simulink model "R0_to_Euler_Test"  (Simulink 7.5)
settings: Solver=ode45  StartTime=0.0  StopTime=10.0  RelTol=1e-3
values from neighbouring files (symbols this model uses):
  R0 = single(Euler2DCMdeg( PHI_IC, THETA_IC, PSI_IC ))    [demoz2SlugsV5.m]
libraries: SLUGS_Library x3, dspmtrx3 x1, simulink x1
settings Model: Creator=Robert  LastModifiedBy=Robert

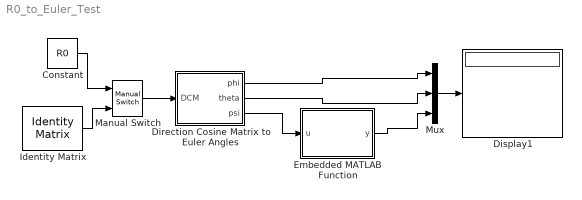
== system R0_to_Euler_Test ==
  Constant : Constant  Value=R0  VectorParams1D=off  OutDataTypeMode=single  OutDataType=fixdt(1, 16)  OutScaling=2^0  OutDataTypeStr=single
  Direction Cosine Matrix to Euler Angles : Subsystem  AncestorBlock=aerolibtransform2/Direction Cosine Matrix to Euler Angles  mask(DCM2Euler){}
      mask help: Determine an euler orientation (roll, pitch, yaw) from the 3-by-3 direction cosine matrix (DCM). The input DCM transforms vectors from geodetic earth or north-down-east (NED) axes to body axes.
      mask init:
      | aeroicon('aeroblk');
      mask Help: web(asbhelp('directioncosinematrixtoeulerangles'));
      mask Display:
      | port_label('output',1,'\phi','texmode','on')
      | port_label('output',2,'\theta','texmode','on')
      | port_label('output',3,'\psi','texmode','on')
      | port_label('input',1,'DCM_{be}','texmode','on')
  Display1 : Display
  Embedded MATLAB Function : Stateflow chart  TreatAsAtomicUnit=on
  Identity Matrix : dspmtrx3/Identity Matrix  Inherit=off  N=3  Ts=-1  dataType=single  isSigned=on  wordLen=16  udDataType=sfix(16)  fracBitsMode=Best precision  numFracBits=15
  Manual Switch : simulink/Signal Routing/Manual Switch  SystemSampleTime=-1  sw=1  action=0  varsize=off
  Mux : Mux  Inputs=3
  wires:
  Embedded MATLAB Function/1(y) -> Mux/3
  Direction Cosine Matrix to Euler Angles/2(theta) -> Mux/2
  Direction Cosine Matrix to Euler Angles/1(phi) -> Mux/1
  Direction Cosine Matrix to Euler Angles/3(psi) -> Embedded MATLAB Function/1(u)
  Mux/1 -> Display1/1
  Constant/1 -> Manual Switch/1
  Manual Switch/1 -> Direction Cosine Matrix to Euler Angles/1(DCM)
  Identity Matrix/1 -> Manual Switch/2

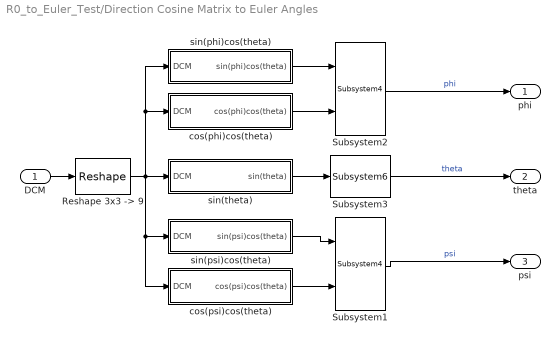
== system R0_to_Euler_Test/Direction Cosine Matrix to Euler Angles ==
  DCM : Inport  PortDimensions=[3,3]  OutDataType=sfix(16)  OutScaling=2^0
  "Reshape 3x3 -> 9" : Reshape  OutputDimensions=[9, 1]
  Subsystem1 : SLUGS_Library/Subsystem4  SystemSampleTime=-1
  Subsystem2 : SLUGS_Library/Subsystem4  SystemSampleTime=-1
  Subsystem3 : SLUGS_Library/Subsystem6  SystemSampleTime=-1
  cos(phi)cos(theta) : Subsystem
  cos(psi)cos(theta) : Subsystem
  sin(phi)cos(theta) : Subsystem
  sin(psi)cos(theta) : Subsystem
  sin(theta) : Subsystem
  phi : Outport  PortDimensions=1  OutDataType=sfix(16)  OutScaling=2^0  InitialOutput=0
  theta : Outport  Port=2  PortDimensions=1  OutDataType=sfix(16)  OutScaling=2^0  InitialOutput=0
  psi : Outport  Port=3  PortDimensions=1  OutDataType=sfix(16)  OutScaling=2^0  InitialOutput=0
  wires:
  DCM/1 -> "Reshape 3x3 -> 9"/1
  "Reshape 3x3 -> 9"/1 -> sin(theta)/1(DCM), cos(phi)cos(theta)/1(DCM), sin(phi)cos(theta)/1(DCM), cos(psi)cos(theta)/1(DCM), sin(psi)cos(theta)/1(DCM)
  sin(theta)/1(sin(theta)) -> Subsystem3/1
  sin(phi)cos(theta)/1(sin(phi)cos(theta)) -> Subsystem2/1
  cos(phi)cos(theta)/1(cos(phi)cos(theta)) -> Subsystem2/2
  sin(psi)cos(theta)/1(sin(psi)cos(theta)) -> Subsystem1/1
  cos(psi)cos(theta)/1(cos(psi)cos(theta)) -> Subsystem1/2
  Subsystem2/1 -> phi/1  "phi"
  Subsystem3/1 -> theta/1  "theta"
  Subsystem1/1 -> psi/1  "psi"

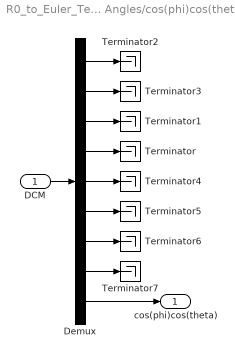
== system R0_to_Euler_Test/Direction Cosine Matrix to Euler Angles/cos(phi)cos(theta) ==
  DCM : Inport  OutDataType=sfix(16)  OutScaling=2^0
  Demux : Demux  Outputs=9
  Terminator{,1..7} (8 alike) : Terminator
  cos(phi)cos(theta) : Outport  OutDataType=sfix(16)  OutScaling=2^0
  wires:
  Demux/4 -> Terminator/1
  Demux/3 -> Terminator1/1
  Demux/5 -> Terminator4/1
  Demux/2 -> Terminator3/1
  Demux/1 -> Terminator2/1
  DCM/1 -> Demux/1
  Demux/8 -> Terminator7/1
  Demux/6 -> Terminator5/1
  Demux/7 -> Terminator6/1
  Demux/9 -> cos(phi)cos(theta)/1

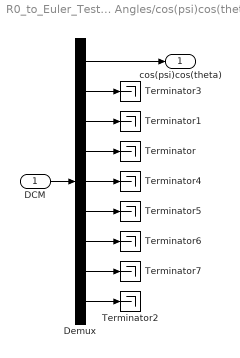
== system R0_to_Euler_Test/Direction Cosine Matrix to Euler Angles/cos(psi)cos(theta) ==
  DCM : Inport  OutDataType=sfix(16)  OutScaling=2^0
  Demux : Demux  Outputs=9
  Terminator{,1..7} (8 alike) : Terminator
  cos(psi)cos(theta) : Outport  OutDataType=sfix(16)  OutScaling=2^0
  wires:
  Demux/9 -> Terminator2/1
  Demux/7 -> Terminator6/1
  Demux/6 -> Terminator5/1
  Demux/8 -> Terminator7/1
  DCM/1 -> Demux/1
  Demux/1 -> cos(psi)cos(theta)/1
  Demux/2 -> Terminator3/1
  Demux/5 -> Terminator4/1
  Demux/3 -> Terminator1/1
  Demux/4 -> Terminator/1

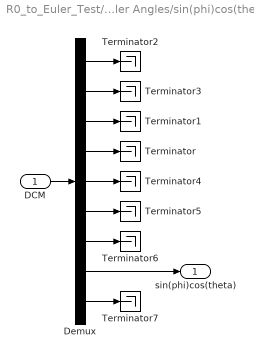
== system R0_to_Euler_Test/Direction Cosine Matrix to Euler Angles/sin(phi)cos(theta) ==
  DCM : Inport  OutDataType=sfix(16)  OutScaling=2^0
  Demux : Demux  Outputs=9
  Terminator{,1..7} (8 alike) : Terminator
  sin(phi)cos(theta) : Outport  OutDataType=sfix(16)  OutScaling=2^0
  wires:
  Demux/9 -> Terminator7/1
  Demux/7 -> Terminator6/1
  Demux/6 -> Terminator5/1
  Demux/8 -> sin(phi)cos(theta)/1
  DCM/1 -> Demux/1
  Demux/1 -> Terminator2/1
  Demux/2 -> Terminator3/1
  Demux/5 -> Terminator4/1
  Demux/3 -> Terminator1/1
  Demux/4 -> Terminator/1

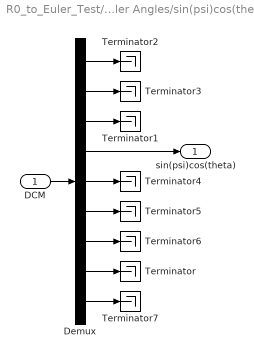
== system R0_to_Euler_Test/Direction Cosine Matrix to Euler Angles/sin(psi)cos(theta) ==
  DCM : Inport  OutDataType=sfix(16)  OutScaling=2^0
  Demux : Demux  Outputs=9
  Terminator{,1..7} (8 alike) : Terminator
  sin(psi)cos(theta) : Outport  OutDataType=sfix(16)  OutScaling=2^0
  wires:
  Demux/4 -> sin(psi)cos(theta)/1
  Demux/3 -> Terminator1/1
  Demux/5 -> Terminator4/1
  Demux/2 -> Terminator3/1
  Demux/1 -> Terminator2/1
  DCM/1 -> Demux/1
  Demux/8 -> Terminator/1
  Demux/6 -> Terminator5/1
  Demux/7 -> Terminator6/1
  Demux/9 -> Terminator7/1

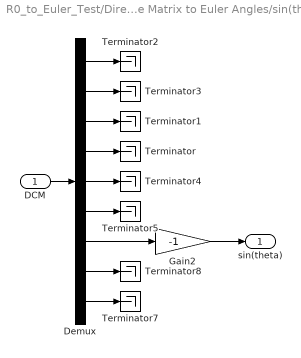
== system R0_to_Euler_Test/Direction Cosine Matrix to Euler Angles/sin(theta) ==
  DCM : Inport  OutDataType=sfix(16)  OutScaling=2^0
  Demux : Demux  Outputs=9
  Gain2 : Gain  Gain=-1  ParameterDataType=sfix(16)  ParameterScaling=2^0  OutDataType=sfix(16)  OutScaling=2^0  SaturateOnIntegerOverflow=on  OutDataTypeStr=Inherit: Same as input  ParamDataTypeStr=Inherit: Same as input
  Terminator{,1..5,7..8} (8 alike) : Terminator
  sin(theta) : Outport  OutDataType=sfix(16)  OutScaling=2^0
  wires:
  Gain2/1 -> sin(theta)/1
  Demux/4 -> Terminator/1
  Demux/3 -> Terminator1/1
  Demux/5 -> Terminator4/1
  Demux/2 -> Terminator3/1
  Demux/1 -> Terminator2/1
  DCM/1 -> Demux/1
  Demux/8 -> Terminator8/1
  Demux/6 -> Terminator5/1
  Demux/7 -> Gain2/1
  Demux/9 -> Terminator7/1

== matlab function Embedded MATLAB Function ==
  data: u input double; y output double
function y = TwoPi(u)
% This block supports an embeddable subset of the MATLAB language.
% See the help menu for details. 

if ( u < 0 )
    y = u + 2*pi;
else
    y = u;
end
